simulink model "QuadruppelTank_BarDyn"  (R2023b)
settings: Solver=VariableStepAuto  StartTime=0.0  StopTime=simu.T_end  RelTol=1e-5
values from neighbouring files (symbols this model uses):
  sys = []    [mainSimulation_bar.m]
undefined symbols (not defined in the file or in its folder): simu
libraries: simulink x4
settings Model: Creator=20155555  LastModifiedBy=20155555

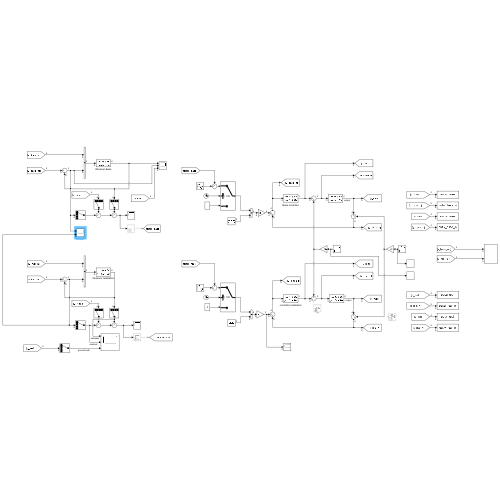
[thumbnail: Simulink's stored preview of the top-level diagram]
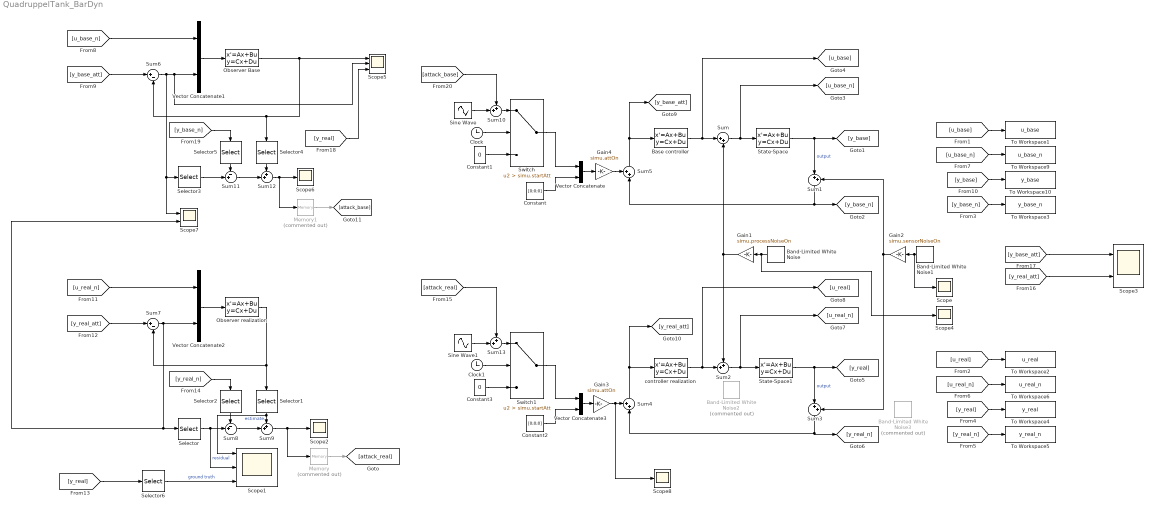
== system QuadruppelTank_BarDyn ==
  Band-Limited White Noise : simulink/Sources/Band-Limited White Noise  Cov=simu.noisePower_input  Ts=simu.dt  seed=[23341]
  Band-Limited White Noise1 : simulink/Sources/Band-Limited White Noise  Cov=simu.noisePower_output  Ts=simu.dt  seed=[23341]
  Band-Limited White Noise2 : simulink/Sources/Band-Limited White Noise  Commented=on  Cov=simu.noisePower_input  Ts=simu.dt  seed=[23341]
  Band-Limited White Noise3 : simulink/Sources/Band-Limited White Noise  Commented=on  Cov=simu.noisePower_output  Ts=simu.dt  seed=[23341]
  Base controller : StateSpace  A=sys.Ac  B=sys.Bc  C=sys.Cc  D=sys.Dc  InitialCondition=simu.rho_0
  Clock : Clock
  Clock1 : Clock
  Constant : Constant  Value=[0;0;0]
  Constant1 : Constant  Value=0
  Constant2 : Constant  Value=[0;0;0]
  Constant3 : Constant  Value=0
  Gain1 : Gain  Gain=simu.processNoiseOn
  Gain2 : Gain  Gain=simu.sensorNoiseOn
  Gain3 : Gain  Gain=simu.attOn
  Gain4 : Gain  Gain=simu.attOn
  Memory : Memory  Commented=on  InheritSampleTime=on
  Memory1 : Memory  Commented=on  InheritSampleTime=on
  Observer Base : StateSpace  A=sys.A  B=[sys.B, sys.L]  C=sys.C  D=zeros(4,6)  InitialCondition=simu.x0_obs  ParameterTunability=Optimized
  Observer realization : StateSpace  A=sys.A  B=[sys.B, sys.L]  C=sys.C  D=zeros(4,6)  InitialCondition=simu.x0_obs  ParameterTunability=Optimized
  Scope{,2,4,6,8} (5 alike) : Scope
  Scope1 : Scope  NumInputPorts=3
  Scope3 : Scope  NumInputPorts=2
  Scope5 : Scope  NumInputPorts=3
  Scope7 : Scope  NumInputPorts=2
  Selector{,1..6} (7 alike) : Selector  InputPortWidth=4  IndexOptions=Index vector (dialog)  Indices=[1 ]  OutputSizes=1
  Sine Wave : Sin  Amplitude=simu.attAmp  Frequency=simu.attFreq  SampleTime=0
  Sine Wave1 : Sin  Amplitude=simu.attAmp  Frequency=simu.attFreq  SampleTime=simu.dt
  State-Space : StateSpace  A=sys.A  B=sys.B  C=sys.C  D=sys.D  InitialCondition=simu.x0_bar  ParameterTunability=Unconstrained
  State-Space1 : StateSpace  A=sys.A  B=sys.B  C=sys.C  D=sys.D  InitialCondition=simu.x0_bar  ParameterTunability=Unconstrained
  Sum : Sum  Inputs=|++
  Sum1 : Sum  Inputs=|++
  Sum{2,4..5,9..10,12..13} (7 alike) : Sum  Inputs=++|
  Sum11 : Sum  Inputs=-+|
  Sum3 : Sum  Inputs=|++
  Sum6 : Sum  Inputs=|+-
  Sum7 : Sum  Inputs=|+-
  Sum8 : Sum  Inputs=-+|
  Switch : Switch  Criteria=u2 > Threshold  Threshold=simu.startAtt  SaturateOnIntegerOverflow=off  InputSameDT=off
  Switch1 : Switch  Criteria=u2 > Threshold  Threshold=simu.startAtt  SaturateOnIntegerOverflow=off  InputSameDT=off
  To Workspace1 : ToWorkspace  VariableName=u_base  SampleTime=-1
      settings: Save2DSignal=2-D array (concatenate along first dimension)
  To Workspace10 : ToWorkspace  VariableName=y_base  SampleTime=-1
      settings: Save2DSignal=2-D array (concatenate along first dimension)
  To Workspace2 : ToWorkspace  VariableName=u_real  SampleTime=-1
      settings: Save2DSignal=2-D array (concatenate along first dimension)
  To Workspace3 : ToWorkspace  VariableName=y_base_n  SampleTime=-1
      settings: Save2DSignal=2-D array (concatenate along first dimension)
  To Workspace4 : ToWorkspace  VariableName=y_real  SampleTime=-1
      settings: Save2DSignal=2-D array (concatenate along first dimension)
  To Workspace5 : ToWorkspace  VariableName=y_real_n  SampleTime=-1
      settings: Save2DSignal=2-D array (concatenate along first dimension)
  To Workspace6 : ToWorkspace  VariableName=u_real_n  SampleTime=-1
      settings: Save2DSignal=2-D array (concatenate along first dimension)
  To Workspace9 : ToWorkspace  VariableName=u_base_n  SampleTime=-1
      settings: Save2DSignal=2-D array (concatenate along first dimension)
  Vector Concatenate{,1..3} (4 alike) : Concatenate
  controller realization : StateSpace  A=sys.Ac_F  B=sys.Bc_F  C=sys.Cc_F  D=sys.Dc_F  InitialCondition=simu.rhoF_0
  wires:
  [u_base_n] -> To Workspace9/1
  [y_base] -> To Workspace10/1
  State-Space/1 -> Sum1/1, [y_base]  "output"
  Sum1/1 -> Sum5/2, [y_base_n]
  Base controller/1 -> [u_base], Sum/1
  Sum/1 -> [u_base_n], State-Space/1
  [u_base] -> To Workspace1/1
  [y_base_n] -> To Workspace3/1
  State-Space1/1 -> Sum3/1, [y_real]  "output"
  [y_real] -> To Workspace4/1
  [u_real_n] -> To Workspace6/1
  controller realization/1 -> [u_real], Sum2/2
  [u_real] -> To Workspace2/1
  Sum2/1 -> [u_real_n], State-Space1/1
  [y_real_n] -> To Workspace5/1
  Sum3/1 -> Sum4/2, [y_real_n]
  Sum4/1 -> [y_real_att], controller realization/1
  Sum5/1 -> [y_base_att], Base controller/1
  Constant/1 -> Vector Concatenate/2
  Constant1/1 -> Switch/3
  Clock/1 -> Switch/2
  Switch/1 -> Vector Concatenate/1
  Vector Concatenate2/1 -> Observer realization/1
  [u_real_n] -> Vector Concatenate2/1
  Observer realization/1 -> Selector1/1, Sum7/2
  Sum7/1 -> Vector Concatenate2/2, Scope7/2, Selector/1
  [y_real_att] -> Sum7/1
  Selector/1 -> Sum8/2, Scope1/2  "residual"
  Sum8/1 -> Sum9/2
  Selector1/1 -> Scope1/1, Sum9/1  "estimate"
  [y_real_n] -> Selector2/1
  Selector2/1 -> Sum8/1
  Sum10/1 -> Switch/1
  Sine Wave/1 -> Sum10/2
  [y_real_att] -> Scope3/2
  [y_base_att] -> Scope3/1
  Sum11/1 -> Sum12/2
  [y_real] -> Scope5/3
  [y_base_att] -> Sum6/1
  Sum6/1 -> Scope7/1, Selector3/1, Scope5/2, Vector Concatenate1/2
  Observer Base/1 -> Scope5/1, Selector4/1, Sum6/2
  Vector Concatenate1/1 -> Observer Base/1
  [u_base_n] -> Vector Concatenate1/1
  Selector3/1 -> Sum11/2
  [y_base_n] -> Selector5/1
  Selector4/1 -> Sum12/1
  Selector5/1 -> Sum11/1
  Switch1/1 -> Vector Concatenate3/1
  Constant3/1 -> Switch1/3
  Constant2/1 -> Vector Concatenate3/2
  Clock1/1 -> Switch1/2
  Sum13/1 -> Switch1/1
  Sine Wave1/1 -> Sum13/2
  Sum12/1 -> Memory1/1, Scope6/1
  Sum9/1 -> Scope2/1, Memory/1
  Vector Concatenate/1 -> Gain4/1
  Vector Concatenate3/1 -> Gain3/1
  Band-Limited White Noise/1 -> Scope4/1, Gain1/1
  Gain1/1 -> Sum/2, Sum2/1
  Gain2/1 -> Sum3/2, Sum1/2
  Band-Limited White Noise1/1 -> Scope/1, Gain2/1
  Gain3/1 -> Scope8/1, Sum4/1
  Gain4/1 -> Sum5/1
  Memory/1 -> [attack_real]
  Memory1/1 -> [attack_base]
  [attack_real] -> Sum13/1
  [attack_base] -> Sum10/1
  [y_real] -> Selector6/1
  Selector6/1 -> Scope1/3  "ground truth"
